simulink model "penduloInvNoLinealV2"  (Simulink 7.9)
settings: Solver=ode45  StartTime=0.0  StopTime=100  RelTol=1e-3
settings Model: Creator=root  LastModifiedBy=root

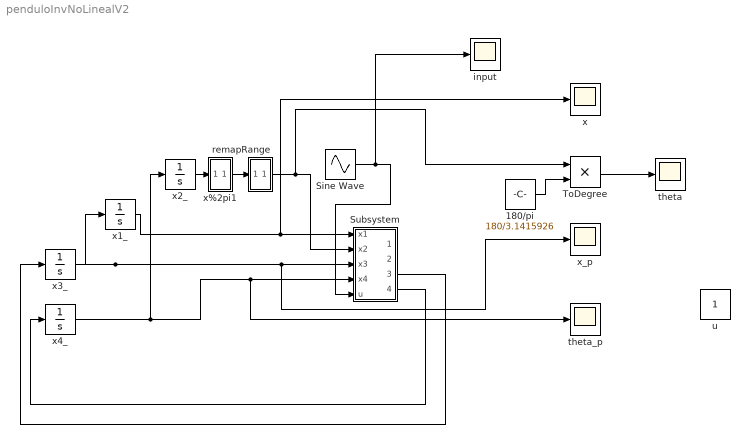
== system penduloInvNoLinealV2 ==
  180/pi : Constant  Value=180/3.1415926
  Sine Wave : Sin  Amplitude=5  Frequency=10
  Subsystem : Subsystem
  ToDegree : Product  RndMeth=Zero
  input : Scope
      settings: SaveName=ScopeData4
  remapRange : MATLAB Function  TreatAsAtomicUnit=on
  theta : Scope
      settings: SaveName=theta
  theta_p : Scope
      settings: SaveName=ScopeData3
  u : Constant
  x : Scope
  x%2pi1 : MATLAB Function  TreatAsAtomicUnit=on
  x1_ : Integrator  UpperSaturationLimit=100  LowerSaturationLimit=-100
  x2_ : Integrator  InitialCondition=pi/2  UpperSaturationLimit=2*pi  LowerSaturationLimit=0
  x3_ : Integrator  UpperSaturationLimit=100  LowerSaturationLimit=-100
  x4_ : Integrator  UpperSaturationLimit=100  LowerSaturationLimit=-100
  x_p : Scope
      settings: SaveName=ScopeData2
  wires:
  Sine Wave/1 -> Subsystem/5(u), input/1
  Subsystem/3(phi3) -> x3_/1
  Subsystem/4(phi4) -> x4_/1
  x3_/1 -> x_p/1, Subsystem/3(x3), x1_/1
  x4_/1 -> theta_p/1, Subsystem/4(x4), x2_/1
  180/pi/1 -> ToDegree/2
  ToDegree/1 -> theta/1
  x1_/1 -> Subsystem/1(x1), x/1
  remapRange/1(y) -> Subsystem/2(x2), ToDegree/1
  x2_/1 -> x%2pi1/1(u)
  x%2pi1/1(y) -> remapRange/1(value)

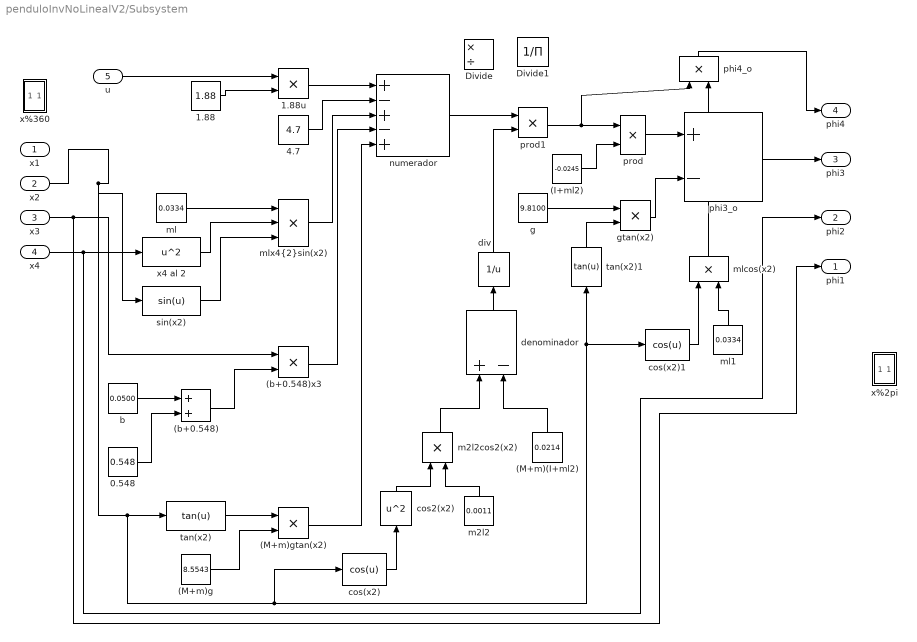
== system penduloInvNoLinealV2/Subsystem ==
  x1 : Inport
  x2 : Inport  Port=2
  x3 : Inport  Port=3
  x4 : Inport  Port=4
  u : Inport  Port=5
  (I+ml2) : Constant  Value=-0.0245
  (M+m)(I+ml2) : Constant  Value=0.0214
  (M+m)g : Constant  Value=8.5543
  (M+m)gtan(x2) : Product  RndMeth=Zero
  (b+0.548) : Sum
  (b+0.548)x3 : Product  RndMeth=Zero
  0.548 : Constant  Value=0.548
  1.88 : Constant  Value=1.88
  1.88u : Product  RndMeth=Zero
  4.7 : Constant  Value=4.7
  Divide : Product  Inputs=*/
  Divide1 : Product  Inputs=/
  b : Constant  Value=0.0500
  cos(x2) : Fcn  Expr=cos(u)  SampleTime=0.1
  cos(x2)1 : Fcn  Expr=cos(u)  SampleTime=0.1
  cos2(x2) : Fcn  Expr=u^2  SampleTime=0.1
  denominador : Sum  Inputs=+-
  div : Fcn  Expr=1/u  SampleTime=0.1
  g : Constant  Value=9.8100
  gtan(x2) : Product  RndMeth=Zero
  m2l2 : Constant  Value=0.0011
  m2l2cos2(x2) : Product  RndMeth=Zero
  ml : Constant  Value=0.0334
  ml1 : Constant  Value=0.0334
  mlcos(x2) : Product  RndMeth=Zero
  "mlx4{2}sin(x2)" : Product  Inputs=3  RndMeth=Zero
  numerador : Sum  Inputs=+-+-+
  phi3_o : Sum  Inputs=+-
  phi4_o : Product  RndMeth=Zero
  prod : Product  RndMeth=Zero
  prod1 : Product  RndMeth=Zero
  sin(x2) : Fcn  Expr=sin(u)  SampleTime=0.1
  tan(x2) : Fcn  Expr=tan(u)  SampleTime=0.1
  tan(x2)1 : Fcn  Expr=tan(u)  SampleTime=0.1
  x%2pi : MATLAB Function  TreatAsAtomicUnit=on
  x%360 : MATLAB Function  TreatAsAtomicUnit=on
  x4 al 2 : Fcn  Expr=u^2  SampleTime=0.1
  phi1 : Outport
  phi2 : Outport  Port=2
  phi3 : Outport  Port=3
  phi4 : Outport  Port=4
  wires:
  1.88/1 -> 1.88u/2
  u/1 -> 1.88u/1
  1.88u/1 -> numerador/1
  4.7/1 -> numerador/2
  ml/1 -> "mlx4{2}sin(x2)"/1
  sin(x2)/1 -> "mlx4{2}sin(x2)"/3
  x4 al 2/1 -> "mlx4{2}sin(x2)"/2
  x4/1 -> x4 al 2/1, phi2/1
  "mlx4{2}sin(x2)"/1 -> numerador/3
  (b+0.548)x3/1 -> numerador/4
  x3/1 -> (b+0.548)x3/1, phi1/1
  (b+0.548)/1 -> (b+0.548)x3/2
  b/1 -> (b+0.548)/1
  0.548/1 -> (b+0.548)/2
  (M+m)gtan(x2)/1 -> numerador/5
  tan(x2)/1 -> (M+m)gtan(x2)/1
  (M+m)g/1 -> (M+m)gtan(x2)/2
  (M+m)(I+ml2)/1 -> denominador/2
  m2l2cos2(x2)/1 -> denominador/1
  cos2(x2)/1 -> m2l2cos2(x2)/1
  m2l2/1 -> m2l2cos2(x2)/2
  cos(x2)/1 -> cos2(x2)/1
  numerador/1 -> prod1/1
  prod1/1 -> prod/1, phi4_o/1
  (I+ml2)/1 -> prod/2
  prod/1 -> phi3_o/1
  gtan(x2)/1 -> phi3_o/2
  g/1 -> gtan(x2)/1
  tan(x2)1/1 -> gtan(x2)/2
  mlcos(x2)/1 -> phi4_o/2
  ml1/1 -> mlcos(x2)/2
  cos(x2)1/1 -> mlcos(x2)/1
  phi3_o/1 -> phi3/1
  phi4_o/1 -> phi4/1
  denominador/1 -> div/1
  div/1 -> prod1/2
  x2/1 -> sin(x2)/1, tan(x2)/1, cos(x2)/1, tan(x2)1/1, cos(x2)1/1

== matlab function Subsystem/x%2pi ==
  data: u input double; y output double
function y = fcn(u)
%#codegen

    y = mod(u,2*pi);
end

== matlab function Subsystem/x%360 ==
  data: u input double; y output double
function y = fcn(u)
%#codegen

    y = mod(u,2*pi);
end

== matlab function remapRange ==
  data: value input double; y output double
function y = remapRange(value)
    scaleFactor = pi/180;
    if (value>180*scaleFactor)
        %constants
        fromLow = 181*scaleFactor;
        fromHigh = 360*scaleFactor;
        toLow = -179*scaleFactor;
        toHigh = 0*scaleFactor;
        %calculations
        new_range = toHigh-toLow;
        old_range = fromHigh - fromLow;
        new_value = (new_range/old_range)*(value-fromLow)+toLow;
        y = new_value;
    else
        y = value;
    end
        
end

== matlab function x%2pi1 ==
  data: u input double; y output double
function y = fcn(u)
%#codegen

    y = mod(u,2*pi);
end
